simulink model "actual_04_constant_measured"  (R2024b)
settings: Solver=VariableStepAuto  StartTime=0.0  StopTime=5.4  RelTol=1e-3
model workspace (MAT data in the model file):
  position_data = timeseries
  position_data.Name = 'unnamed'
  position_data.DataInfo = tsdata.datametadata
  position_data.DataInfo.Interpolation = tsdata.interpolation
  position_data.DataInfo.Interpolation.Fhandle : function handle (value not decoded)
  position_data.DataInfo.Interpolation.Name = 'linear'
  position_data.TimeInfo = tsdata.timemetadata
  position_data.TimeInfo.Length = 54
  position_data.TimeInfo.DuplicateTimes = 0
  position_data.TimeInfo.Time_ = [0.1; 0.2; 0.3; 0.4; 0.5; 0.6; 0.7; 0.8; 0.9; 1; 1.1; 1.2; 1.3; 1.4; 1.5; 1.6; 1.7; 1.8; 1.9; 2; 2.1; 2.2; 2.3; 2.4; 2.5; 2.6; 2.7; 2.8; 2.9; 3; 3.1; 3.2; 3.3; 3.4; 3.5; 3.6; 3.7; 3.8; 3.9; 4; 4.1; 4.2; 4.3; 4.4; 4.5; 4.6; 4.7; 4.8; 4.9; 5; 5.1; 5.2; 5.3; 5.4]
  position_data.TimeInfo.Initialized = 1
  position_data.QualityInfo = tsdata.qualmetadata
  position_data.Data_ = [0; 59.68; 70.27; 32.73; 32.73; 51.98; 51.98; 47.17; 46.2; 46.2; 46.2; 46.2; 46.2; 46.2; 46.2; 46.2; 46.2; 46.2; 46.2; 46.2; 46.2; 46.2; 46.2; 46.2; 46.2; 46.2; 46.2; 46.2; 46.2; 46.2; 46.2; 46.2; 46.2; 46.2; 46.2; 46.2; 46.2; 46.2; 46.2; 46.2; 46.2; 46.2; 46.2; 46.2; 46.2; 46.2; 46.2; 46.2; 46.2; 46.2; 46.2; 46.2; 46.2; 46.2]
  reference_data = timeseries
  reference_data.Name = 'unnamed'
  reference_data.DataInfo = tsdata.datametadata
  reference_data.DataInfo.Interpolation = tsdata.interpolation
  reference_data.DataInfo.Interpolation.Fhandle : function handle (value not decoded)
  reference_data.DataInfo.Interpolation.Name = 'linear'
  reference_data.TimeInfo = tsdata.timemetadata
  reference_data.TimeInfo.Length = 54
  reference_data.TimeInfo.DuplicateTimes = 0
  reference_data.TimeInfo.Time_ = [0.1; 0.2; 0.3; 0.4; 0.5; 0.6; 0.7; 0.8; 0.9; 1; 1.1; 1.2; 1.3; 1.4; 1.5; 1.6; 1.7; 1.8; 1.9; 2; 2.1; 2.2; 2.3; 2.4; 2.5; 2.6; 2.7; 2.8; 2.9; 3; 3.1; 3.2; 3.3; 3.4; 3.5; 3.6; 3.7; 3.8; 3.9; 4; 4.1; 4.2; 4.3; 4.4; 4.5; 4.6; 4.7; 4.8; 4.9; 5; 5.1; 5.2; 5.3; 5.4]
  reference_data.TimeInfo.Initialized = 1
  reference_data.QualityInfo = tsdata.qualmetadata
  reference_data.Data_ = [45; 45; 45; 45; 45; 45; 45; 45; 45; 45; 45; 45; 45; 45; 45; 45; 45; 45; 45; 45; 45; 45; 45; 45; 45; 45; 45; 45; 45; 45; 45; 45; 45; 45; 45; 45; 45; 45; 45; 45; 45; 45; 45; 45; 45; 45; 45; 45; 45; 45; 45; 45; 45; 45]
settings Model: Creator=santi  LastModifiedBy=santi

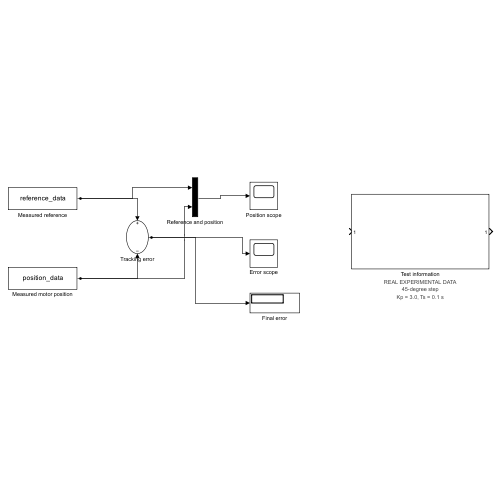
[thumbnail: Simulink's stored preview of the top-level diagram]
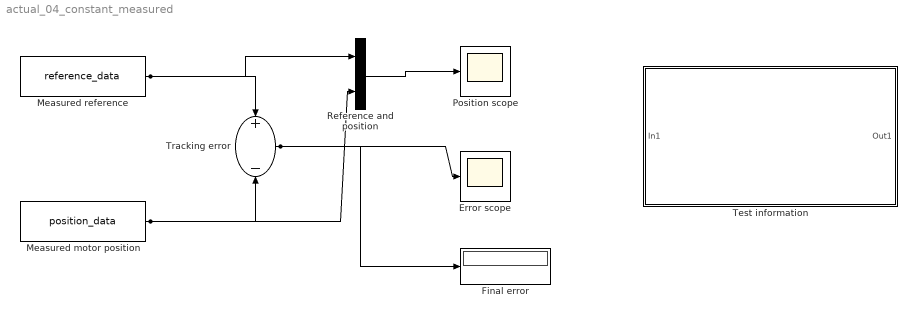
== system actual_04_constant_measured ==
  Error scope : Scope
  Final error : Display
  Measured motor position : FromWorkspace  VariableName=position_data
  Measured reference : FromWorkspace  VariableName=reference_data
  Position scope : Scope
  Reference and position : Mux  Inputs=2
  Test information : Subsystem
      settings: AttributesFormatString=|
      | REAL EXPERIMENTAL DATA
      | 45-degree step
      | Kp = 3.0, Ts = 0.1 s
  Tracking error : Sum  Inputs=+-
  wires:
  Measured reference/1 -> Tracking error/1, Reference and position/1
  Measured motor position/1 -> Tracking error/2, Reference and position/2
  Reference and position/1 -> Position scope/1
  Tracking error/1 -> Error scope/1, Final error/1

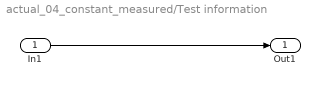
== system actual_04_constant_measured/Test information ==
  In1 : Inport
  Out1 : Outport
  wires:
  In1/1 -> Out1/1
